simulink model "exponential"  (R2024b)
settings: Solver=VariableStepAuto  StartTime=0.0  StopTime=50  RelTol=1e-3
settings Model: Creator=Botló  LastModifiedBy=Botló

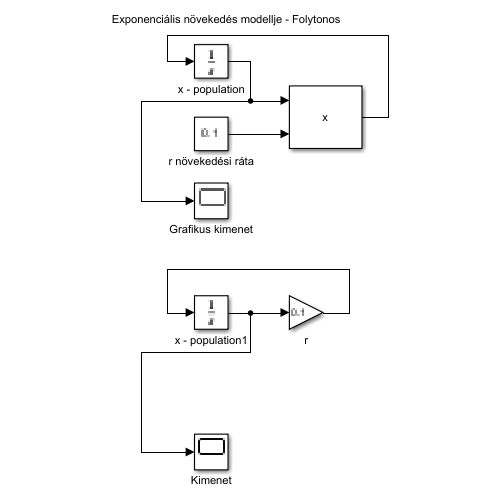
[thumbnail: Simulink's stored preview of the top-level diagram]
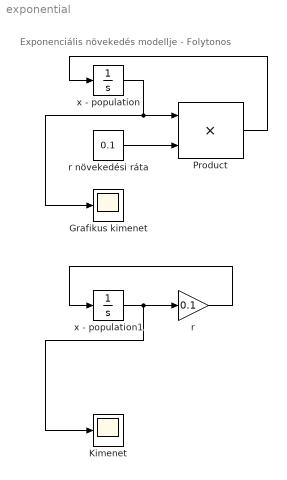
== system exponential ==
  note: Exponenciális növekedés modellje - Folytonos
  Grafikus kimenet : Scope
  Kimenet : Scope
  Product : Product
  r : Gain  Gain=0.1
  r növekedési ráta : Constant  Value=0.1
  x - population : Integrator  InitialCondition=1
  x - population1 : Integrator  InitialCondition=50
  wires:
  r növekedési ráta/1 -> Product/2
  Product/1 -> x - population/1
  x - population/1 -> Grafikus kimenet/1, Product/1
  x - population1/1 -> r/1, Kimenet/1
  r/1 -> x - population1/1
